simulink model "simu3"  (R2024a)
settings: Solver=VariableStepAuto  StartTime=0.0  StopTime=10.0  RelTol=1e-3
settings Model: Creator=psp_dada  LastModifiedBy=psp_dada

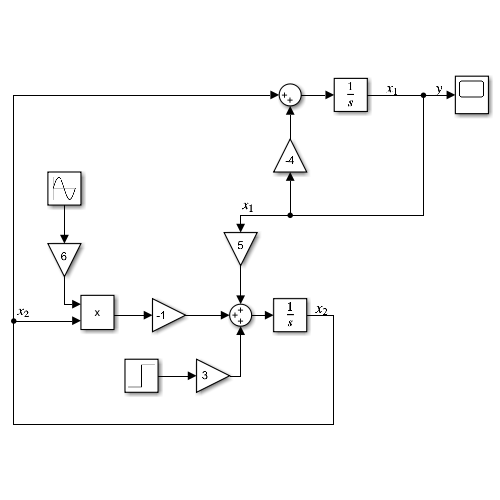
[thumbnail: Simulink's stored preview of the top-level diagram]
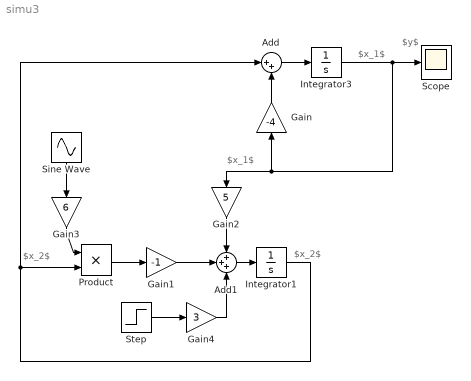
== system simu3 ==
  note: $y$
  note: $x_1$
  note: $x_1$
  note: $x_2$
  note: $x_2$
  Add : Sum  Inputs=|++
  Add1 : Sum  Inputs=+++
  Gain : Gain  Gain=-4
  Gain1 : Gain  Gain=-1
  Gain2 : Gain  Gain=5
  Gain3 : Gain  Gain=6
  Gain4 : Gain  Gain=3
  Integrator1 : Integrator
  Integrator3 : Integrator
  Product : Product
  Scope : Scope
  Sine Wave : Sin  SampleTime=0
  Step : Step  SampleTime=0.001
  wires:
  Gain3/1 -> Product/1
  Integrator1/1 -> Add/1, Product/2
  Gain2/1 -> Add1/1
  Product/1 -> Gain1/1
  Gain4/1 -> Add1/3
  Add/1 -> Integrator3/1
  Integrator3/1 -> Gain2/1, Gain/1, Scope/1
  Add1/1 -> Integrator1/1
  Gain1/1 -> Add1/2
  Gain/1 -> Add/2
  Sine Wave/1 -> Gain3/1
  Step/1 -> Gain4/1
